simulink model "sharedControl2"  (R2018a)
settings: Solver=VariableStepAuto  StartTime=0.0  StopTime=500  RelTol=1e-3
values from neighbouring files (symbols this model uses):
  a = -real(s1) + imag(s1)/tan(angle(s1+b) - theta)    [RLDesignJoystick.m]    (also in gainPlot.m = 10)
  a1 = b1/K    [RLDesignJoystick.m]
  b = 1.2*bb/I    (= 0.4)    [RLDesignJoystick.m]    (also in gainPlot.m)
  b1 = -real(s1)/150    [RLDesignJoystick.m]
  bb = 0.254    [RLDesignJoystick.m]
  I = 0.762    [RLDesignJoystick.m]
  K0 = abs(s1+a)/abs(Gs1)/abs(s1+b)    [RLDesignJoystick.m]    (also in gainPlot.m = 0.5)
  K1 = 1/abs(Gs1)    [RLDesignJoystick.m]
undefined symbols (not defined in the file or in its folder): U
libraries: simulink x1
settings Model: Creator=transmogrifier  LastModifiedBy=transmogrifier
settings SolverCC: ZeroCrossAlgorithm=Adaptive
settings DebuggingCC: MaxConsecutiveZCsMsg=none

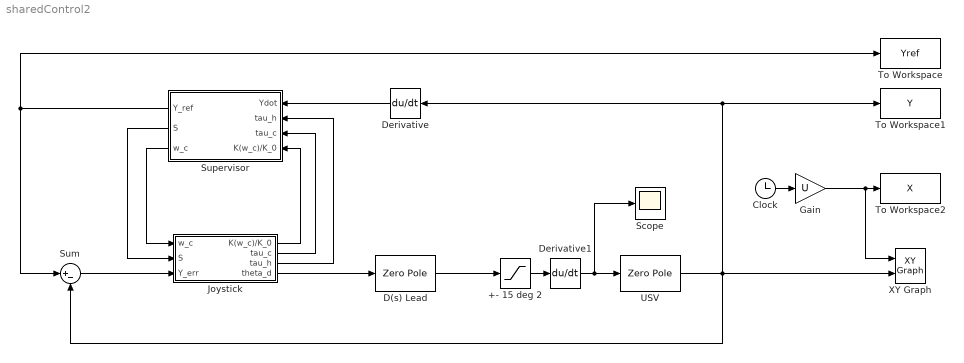
== system sharedControl2 ==
  +- 15 deg 2 : Saturate  UpperLimit=15  LowerLimit=-15
  Clock : Clock
  D(s) Lead : ZeroPole  Zeros=[-.2667]  Poles=[-26.49]  Gain=[1619]
  Derivative : Derivative  CoefficientInTFapproximation=1
  Derivative1 : Derivative
  Gain : Gain  Gain=U
  Joystick : Subsystem  mask{a_d=2, b_d=0.1, tau_h=1.140}
      mask prompts: a_d "a_d used in K(w_das) term"; b_d "b_d used in K(w_das) term"; tau_h "simulated human applied torque"
  Scope : Scope
  Sum : Sum  Inputs=|+-
  Supervisor : Subsystem  mask{S=0, gamma_1_sq=0.1, gamma_2_sq=0.2, sigma_sq=0.3, delta_y=4}
      mask prompts: S "state"; gamma_1_sq "(gamma_1)^2"; gamma_2_sq "(gamma_2)^2"; sigma_sq "sigma^2"; delta_y "lane width"
  To Workspace : ToWorkspace  VariableName=Yref  SaveFormat=Timeseries  SampleTime=-1
  To Workspace1 : ToWorkspace  VariableName=Y  SaveFormat=Timeseries  SampleTime=-1
  To Workspace2 : ToWorkspace  VariableName=X  SaveFormat=Timeseries  SampleTime=-1
  USV : ZeroPole  Zeros=[]  Poles=[0 0 -5/4]  Gain=[U*1e-2]
  XY Graph : simulink/Sinks/XY Graph  xmin=-10  xmax=U*500  ymin=-20  ymax=20  st=-1
  wires:
  Joystick/4(theta_d) -> D(s) Lead/1
  Clock/1 -> Gain/1
  Supervisor/3(w_c) -> Joystick/1(w_c)
  USV/1 -> To Workspace1/1, Derivative/1, XY Graph/2, Sum/2
  Derivative/1 -> Supervisor/1(Ydot)
  Supervisor/1(Y_ref) -> Sum/1, To Workspace/1
  Supervisor/2(S) -> Joystick/2(S)
  Sum/1 -> Joystick/3(Y_err)
  Joystick/2(tau_c) -> Supervisor/3(tau_c)
  Joystick/3(tau_h) -> Supervisor/2(tau_h)
  D(s) Lead/1 -> +- 15 deg 2/1
  Joystick/1(K(w_c)/K_0) -> Supervisor/4(K(w_c)/K_0)
  Gain/1 -> XY Graph/1, To Workspace2/1
  +- 15 deg 2/1 -> Derivative1/1
  Derivative1/1 -> Scope/1, USV/1

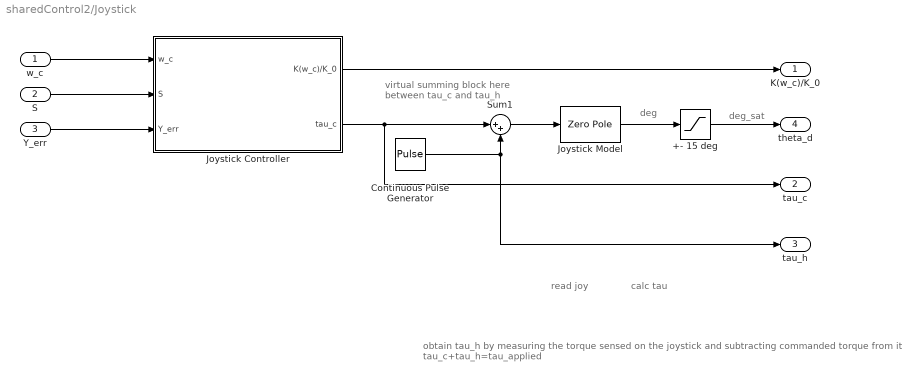
== system sharedControl2/Joystick ==
  note: virtual summing block here
      | between tau_c and tau_h
  note: read joy
  note: obtain tau_h by measuring the torque sensed on the joystick and subtracting commanded torque from it
      | tau_c+tau_h=tau_applied
  note: deg
  note: deg_sat
  note: calc tau
  w_c : Inport
  S : Inport  Port=2
  Y_err : Inport  Port=3
  +- 15 deg : Saturate  UpperLimit=15  LowerLimit=-15
  Continuous Pulse Generator : DiscretePulseGenerator  PulseType=Time based  Amplitude=2  Period=500  PhaseDelay=30
  Joystick Controller : Subsystem
  Joystick Model : ZeroPole  Zeros=[]  Poles=[0 -bb/I]  Gain=[I]
  Sum1 : Sum  Inputs=|++
  K(w_c)/K_0 : Outport
  tau_c : Outport  Port=2
  tau_h : Outport  Port=3
  theta_d : Outport  Port=4
  wires:
  Joystick Model/1 -> +- 15 deg/1
  +- 15 deg/1 -> theta_d/1
  Joystick Controller/2(tau_c) -> Sum1/1, tau_c/1
  Joystick Controller/1(K(w_c)/K_0) -> K(w_c)/K_0/1
  w_c/1 -> Joystick Controller/1(w_c)
  Y_err/1 -> Joystick Controller/3(Y_err)
  Continuous Pulse Generator/1 -> tau_h/1, Sum1/2
  Sum1/1 -> Joystick Model/1
  S/1 -> Joystick Controller/2(S)

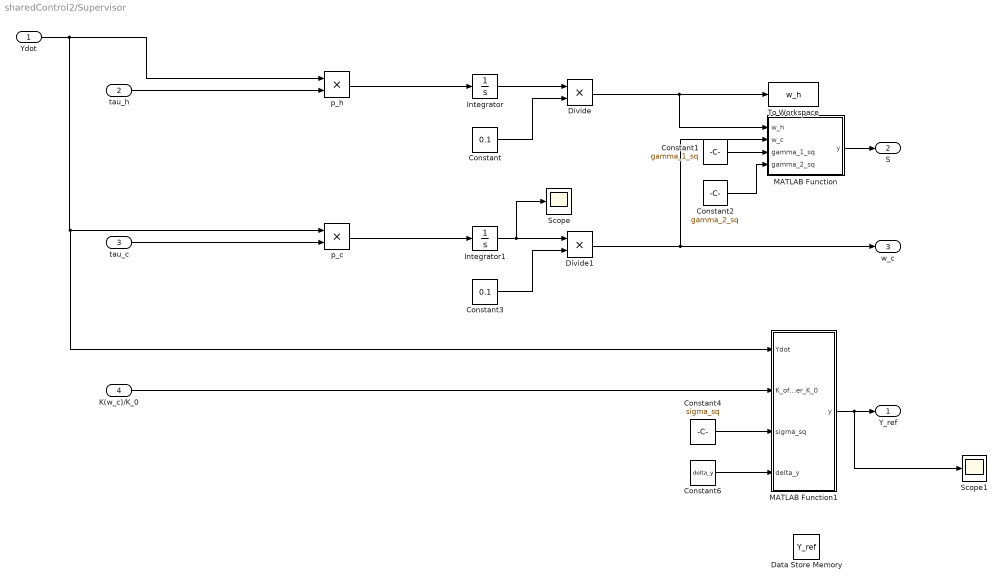
== system sharedControl2/Supervisor ==
  Ydot : Inport
  tau_h : Inport  Port=2
  tau_c : Inport  Port=3
  K(w_c)/K_0 : Inport  Port=4
  Constant : Constant  Value=0.1
  Constant1 : Constant  Value=gamma_1_sq
  Constant2 : Constant  Value=gamma_2_sq
  Constant3 : Constant  Value=0.1
  Constant4 : Constant  Value=sigma_sq
  Constant6 : Constant  Value=delta_y
  Data Store Memory : DataStoreMemory  DataStoreName=Y_ref  ReadBeforeWriteMsg=warning  WriteAfterWriteMsg=warning  WriteAfterReadMsg=warning  ShowAdditionalParam=off  OutDataTypeStr=int16
  Divide : Product
  Divide1 : Product
  Integrator : Integrator  ContinuousStateAttributes='wc'
  Integrator1 : Integrator  ContinuousStateAttributes='wc'
  MATLAB Function : MATLAB Function  TreatAsAtomicUnit=on
  MATLAB Function1 : MATLAB Function  TreatAsAtomicUnit=on
  Scope : Scope
  Scope1 : Scope
  To Workspace : ToWorkspace  VariableName=w_h  SaveFormat=Timeseries  SampleTime=-1
  p_c : Product
  p_h : Product
  Y_ref : Outport
  S : Outport  Port=2
  w_c : Outport  Port=3
  wires:
  Ydot/1 -> MATLAB Function1/1(Ydot), p_c/1, p_h/1
  tau_h/1 -> p_h/2
  p_h/1 -> Integrator/1
  Integrator/1 -> Divide/1
  Constant/1 -> Divide/2
  Divide/1 -> To Workspace/1, MATLAB Function/1(w_h)
  Integrator1/1 -> Scope/1, Divide1/1
  Divide1/1 -> w_c/1, MATLAB Function/2(w_c)
  p_c/1 -> Integrator1/1
  Constant3/1 -> Divide1/2
  tau_c/1 -> p_c/2
  MATLAB Function/1(y) -> S/1
  K(w_c)/K_0/1 -> MATLAB Function1/2(K_of_w_c_over_K_0)
  Constant1/1 -> MATLAB Function/3(gamma_1_sq)
  Constant2/1 -> MATLAB Function/4(gamma_2_sq)
  Constant4/1 -> MATLAB Function1/3(sigma_sq)
  Constant6/1 -> MATLAB Function1/4(delta_y)
  MATLAB Function1/1(y) -> Scope1/1, Y_ref/1

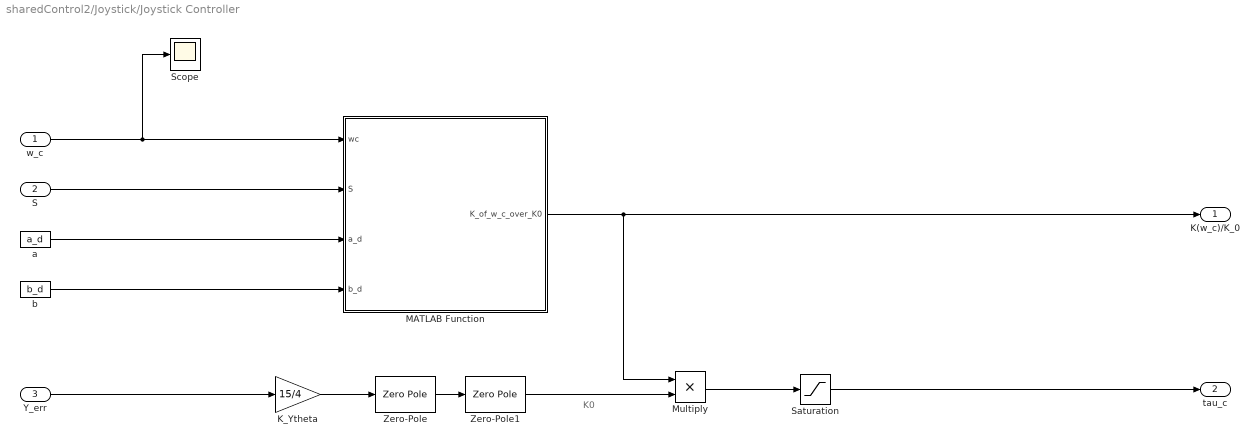
== system sharedControl2/Joystick/Joystick Controller ==
  note: K0
  w_c : Inport
  S : Inport  Port=2
  Y_err : Inport  Port=3
  K_Ytheta : Gain  Gain=15/4
  MATLAB Function : MATLAB Function  TreatAsAtomicUnit=on
  Multiply : Product
  Saturation : Saturate  UpperLimit=3.5  LowerLimit=-3.5
  Scope : Scope
  Zero-Pole : ZeroPole  Zeros=[-b]  Poles=[-a]  Gain=[K0]
  Zero-Pole1 : ZeroPole  Zeros=[-b1]  Poles=[-a1]  Gain=[K1]
  a : Constant  Value=a_d
  b : Constant  Value=b_d
  K(w_c)/K_0 : Outport
  tau_c : Outport  Port=2
  wires:
  Multiply/1 -> Saturation/1
  Y_err/1 -> K_Ytheta/1
  Zero-Pole/1 -> Zero-Pole1/1
  w_c/1 -> Scope/1, MATLAB Function/1(wc)
  a/1 -> MATLAB Function/3(a_d)
  MATLAB Function/1(K_of_w_c_over_K0) -> Multiply/1, K(w_c)/K_0/1
  b/1 -> MATLAB Function/4(b_d)
  Saturation/1 -> tau_c/1
  K_Ytheta/1 -> Zero-Pole/1
  S/1 -> MATLAB Function/2(S)
  Zero-Pole1/1 -> Multiply/2

== matlab function sharedControl2/Supervisor/MATLAB Function ==
  data: w_h input; y output; w_c input; gamma_1_sq input; gamma_2_sq input
function y = fcn(w_h, w_c, gamma_1_sq, gamma_2_sq)

if(w_h >= -gamma_1_sq && w_c >= -gamma_2_sq)
    S=1;
elseif(w_h >= -gamma_1_sq && w_c < -gamma_2_sq)
    S=2;
elseif(w_h < -gamma_1_sq && w_c >= -gamma_2_sq)
    S=3;
elseif(w_h < -gamma_1_sq && w_c < -gamma_2_sq)
    S=4;
else
    error('bad state assignment');
end
y = S;

== matlab function sharedControl2/Joystick/Joystick Controller/MATLAB Function ==
  data: wc input; S input; K_of_w_c_over_K0 output; a_d input; b_d input
function K_of_w_c_over_K0 = fcn(wc, S, a_d, b_d)

if S == 2    
    K_of_w_c_over_K0 = 1/(1 + exp(-a_d*wc + b_d));
else
    K_of_w_c_over_K0 = 1;
end

return

== matlab function sharedControl2/Supervisor/MATLAB Function1 ==
  settings: updateMethod=DISCRETE
  data: Ydot input; y output; K_of_w_c_over_K_0 input; sigma_sq input; delta_y input; Y_ref data_store_memory
function y = fcn(Ydot, K_of_w_c_over_K_0, sigma_sq, delta_y)
%Initial Y_ref, delta_y, and sigma_sq are set in mask)

global Y_ref;

if(K_of_w_c_over_K_0<=sigma_sq)
    if(Ydot<0)
        Y_ref=Y_ref-delta_y;
    elseif(Ydot>0)
        Y_ref=Y_ref+delta_y
    else
        Y_ref=Y_ref;
    end
end

y = Y_ref;
